simulink model "sampleModel2058"  (R2023a)
settings: Solver=VariableStepAuto  StartTime=0.0  StopTime=10.0  RelTol=1e-3
libraries: hdlsllib x4, simulink x2
settings Model: Creator=user1  LastModifiedBy=user1

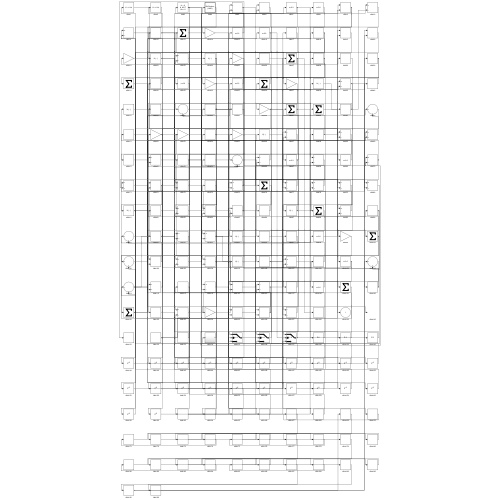
[thumbnail: Simulink's stored preview of the top-level diagram]
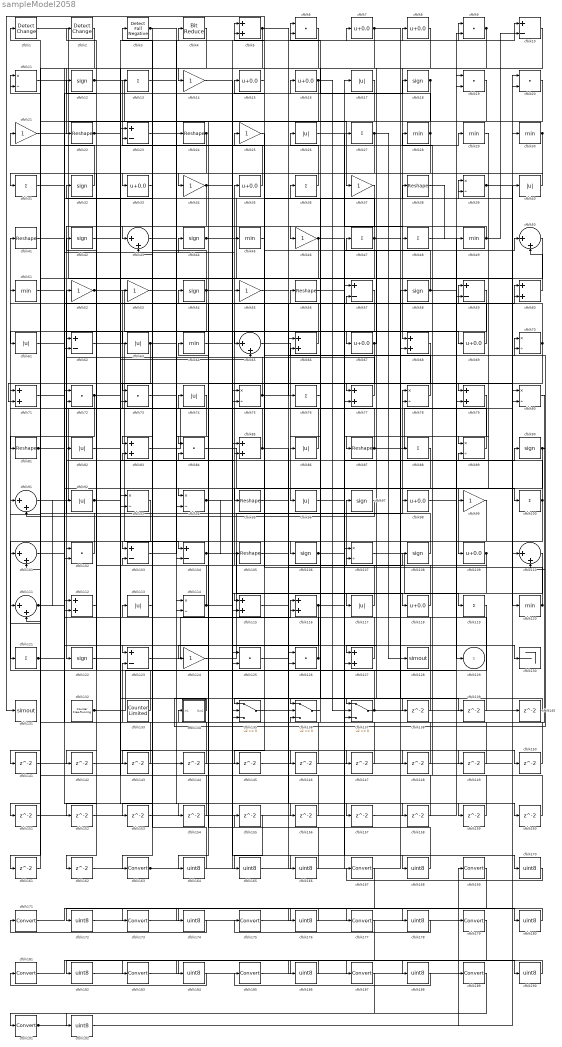
== system sampleModel2058 ==
  cfblk1 : simulink/Logic and Bit Operations/Detect Change  vinit=0  OutDataTypeStr=boolean
      settings: LibrarySourceBlock=|
      | hdlsllib/Logic and Bit
      | Operations/Detect
      | Change
  cfblk{10,23,57,59,62,103..104,123} (8 alike) : Sum  Inputs=+-
  cfblk{13,27,31,36,47..48,76,88,100,119,121} (11 alike) : Sum  Inputs=+
  cfblk{43,50,65,91,101,110..111} (7 alike) : Sum  Inputs=|++
  cfblk{6,9,19..20,72..73,84,102,125..126} (10 alike) : DotProduct  OutDataTypeStr=Inherit: Inherit via internal rule
  cfblk{22,24,38,41,56,81,87,95,105} (9 alike) : Reshape
  cfblk{12,18,32,42,44,54,58,90,97,106,108,122} (12 alike) : Signum
  cfblk{11,39,70,75,78,80,89,93..94,107,114} (11 alike) : Product  Inputs=*/  RndMeth=Zero  SaturateOnIntegerOverflow=on
  cfblk{7..8,15..16,33,35,67,69,98,109,118} (11 alike) : Bias  Bias=0.0  SaturateOnIntegerOverflow=off
  cfblk{5,60,66,68,71,77,79,83,85,112,115..116,127} (13 alike) : Sum
  cfblk{17,26,40,61,63,74,82,86,92,96,113,117} (12 alike) : Abs  SaturateOnIntegerOverflow=off
  cfblk{28..30,45,49,51,64,120} (8 alike) : MinMax
  cfblk{14,21,25,34,37,46,52..53,55,99,124} (11 alike) : Gain
  cfblk128 : ToWorkspace  VariableName=simout  SaveFormat=Timeseries  SampleTime=-1
  cfblk130 : Terminator
  cfblk131 : ToWorkspace  VariableName=simout  SaveFormat=Timeseries  SampleTime=-1
  cfblk132 : hdlsllib/Sources/Counter Free-Running  NumBits=16  tsamp=-1
  cfblk133 : hdlsllib/Sources/Counter Limited  uplimit=7  tsamp=-1
  cfblk134 : Subsystem
      settings: LibrarySourceBlock=|
      | hdlsllib/Ports &
      | Subsystems/Subsystem
  cfblk135 : Switch  SaturateOnIntegerOverflow=off  InputSameDT=off
  cfblk136 : Switch  SaturateOnIntegerOverflow=off  InputSameDT=off
  cfblk137 : Switch  SaturateOnIntegerOverflow=off  InputSameDT=off
  cfblk{138..162} (25 alike) : Delay  SampleTime=1
  cfblk{163,167,169,171,173,175,177,179,181,183,185,187,189,191} (14 alike) : DataTypeConversion  SaturateOnIntegerOverflow=off  RndMeth=Floor
  cfblk{164..166,168,170,172,174,176,178,180,182,184,186,188,190,192} (16 alike) : DataTypeConversion  OutDataTypeStr=uint8  SaturateOnIntegerOverflow=off  RndMeth=Floor
  cfblk2 : simulink/Logic and Bit Operations/Detect Change  vinit=0  OutDataTypeStr=boolean
      settings: LibrarySourceBlock=|
      | hdlsllib/Logic and Bit
      | Operations/Detect
      | Change
  cfblk3 : hdlsllib/Logic and Bit Operations/Detect Fall Negative  vinit=0  OutDataTypeStr=boolean
  cfblk4 : hdlsllib/Logic and Bit Operations/Bit Reduce  mode=AND
  cfblk129 : Outport  VectorParamsAs1DForOutWhenUnconnected=off
  wires:
  cfblk37/1 -> cfblk122/1
  cfblk100/1 -> cfblk102/1, cfblk12/1, cfblk164/1
  cfblk5/1 -> cfblk14/1, cfblk77/1
  cfblk62/1 -> cfblk104/1
  cfblk117/1 -> cfblk35/1
  cfblk25/1 -> cfblk95/1
  cfblk52/1 -> cfblk69/1, cfblk152/1
  cfblk12/1 -> cfblk37/1, cfblk65/2
  cfblk119/1 -> cfblk41/1
  cfblk86/1 -> cfblk15/1
  cfblk89/1 -> cfblk53/1
  cfblk126/1 -> cfblk54/1, cfblk43/2
  cfblk8/1 -> cfblk68/1
  cfblk93/1 -> cfblk121/1
  cfblk113/1 -> cfblk163/1
  cfblk118/1 -> cfblk97/1
  cfblk102/1 -> cfblk52/1
  cfblk57/1 -> cfblk67/1
  cfblk96/1 -> cfblk50/1
  cfblk40/1 -> cfblk34/1
  cfblk84/1 -> cfblk109/1
  cfblk77/1 -> cfblk62/1
  cfblk124/1 -> cfblk78/1
  cfblk123/1 -> cfblk116/1
  cfblk65/1 -> cfblk96/1
  cfblk121/1 -> cfblk56/1, cfblk44/1
  cfblk101/1 -> cfblk16/1
  cfblk51/1 -> cfblk63/1
  cfblk22/1 -> cfblk148/1, cfblk149/1
  cfblk66/1 -> cfblk51/1
  cfblk103/1 -> cfblk59/1
  cfblk21/1 -> cfblk129/1
  cfblk76/1 -> cfblk136/1
  cfblk94/1 -> cfblk105/1, cfblk10/1, cfblk147/1
  cfblk20/1 -> cfblk103/1
  cfblk107/1 -> cfblk119/1
  cfblk114/1 -> cfblk2/1, cfblk150/1
  cfblk115/1 -> cfblk108/1
  cfblk87/1 -> cfblk40/1, cfblk36/1
  cfblk18/1 -> cfblk124/1, cfblk115/2
  cfblk35/1 -> cfblk13/1
  cfblk15/1 -> cfblk131/1
  cfblk1/1 -> cfblk88/1
  cfblk32/1 -> cfblk21/1
  cfblk46/1 -> cfblk101/1, cfblk80/2, cfblk39/1
  cfblk61/1 -> cfblk38/1
  cfblk91/1 -> cfblk68/2
  cfblk85/1 -> cfblk11/1, cfblk158/1
  cfblk60/1 -> cfblk50/2
  cfblk78/1 -> cfblk55/1
  cfblk54/1 -> cfblk32/1, cfblk79/2, cfblk83/1
  cfblk29/1 -> cfblk99/1
  cfblk16/1 -> cfblk31/1, cfblk137/2
  cfblk72/1 -> cfblk111/2, cfblk4/1
  cfblk34/1 -> cfblk6/1, cfblk114/2
  cfblk90/1 -> cfblk112/2, cfblk110/2
  cfblk127/1 -> cfblk82/1
  cfblk81/1 -> cfblk29/1, cfblk45/1
  cfblk38/1 -> cfblk49/1
  cfblk120/1 -> cfblk25/1, cfblk28/1
  cfblk70/1 -> cfblk3/1, cfblk137/1
  cfblk19/1 -> cfblk102/2
  cfblk7/1 -> cfblk46/1, cfblk139/1
  cfblk88/1 -> cfblk106/1
  cfblk98/1 -> cfblk90/1
  cfblk27/1 -> cfblk86/1, cfblk128/1, cfblk75/2
  cfblk112/1 -> cfblk42/1
  cfblk111/1 -> cfblk74/1, cfblk92/1, cfblk157/1
  cfblk83/1 -> cfblk27/1
  cfblk135/1 -> cfblk107/2
  cfblk36/1 -> cfblk26/1
  cfblk41/1 -> cfblk18/1
  cfblk28/1 -> cfblk94/1, cfblk73/2, cfblk6/2
  cfblk80/1 -> cfblk134/1(In1)
  cfblk9/1 -> cfblk93/2, cfblk62/2
  cfblk106/1 -> cfblk98/1, cfblk60/2
  cfblk53/1 -> cfblk24/1
  cfblk24/1 -> cfblk61/1, cfblk161/1
  cfblk110/1 -> cfblk126/2
  cfblk63/1 -> cfblk9/1, cfblk8/1, cfblk71/2
  cfblk108/1 -> cfblk71/1
  cfblk17/1 -> cfblk81/1
  cfblk31/1 -> cfblk123/1
  cfblk134/1(Out1) -> cfblk70/1
  cfblk133/1 -> cfblk91/1
  cfblk33/1 -> cfblk73/1
  cfblk97/1 -> cfblk91/2
  cfblk75/1 -> cfblk23/2, cfblk70/2
  cfblk104/1 -> cfblk117/1, cfblk118/1
  cfblk3/1 -> cfblk77/2, cfblk143/1, cfblk146/1
  cfblk49/1 -> cfblk43/1, cfblk10/2
  cfblk74/1 -> cfblk94/2
  cfblk69/1 -> cfblk11/2
  cfblk39/1 -> cfblk120/1, cfblk89/1
  cfblk6/1 -> cfblk22/1
  cfblk132/1 -> cfblk19/1, cfblk85/1
  cfblk105/1 -> cfblk60/1
  cfblk55/1 -> cfblk76/1
  cfblk50/1 -> cfblk127/1
  cfblk26/1 -> cfblk48/1
  cfblk92/1 -> cfblk130/1, cfblk85/2
  cfblk43/1 -> cfblk104/2
  cfblk44/1 -> cfblk30/1, cfblk80/1, cfblk39/2
  cfblk79/1 -> cfblk127/2
  cfblk67/1 -> cfblk84/1, cfblk47/1
  cfblk11/1 -> cfblk114/1
  cfblk116/1 -> cfblk125/2, cfblk89/2
  cfblk10/1 -> cfblk87/1
  cfblk125/1 -> cfblk57/2
  cfblk4/1 -> cfblk33/1
  cfblk48/1 -> cfblk100/1
  cfblk137/1 -> cfblk72/2, cfblk20/1
  cfblk58/1 -> cfblk19/2, cfblk5/2
  cfblk42/1 -> cfblk79/1
  cfblk109/1 -> cfblk135/3, cfblk103/2
  cfblk45/1 -> cfblk115/1
  cfblk136/1 -> cfblk66/2
  cfblk47/1 -> cfblk59/2, cfblk5/1, cfblk162/1
  cfblk23/1 -> cfblk7/1
  cfblk30/1 -> cfblk65/1, cfblk142/1
  cfblk82/1 -> cfblk138/1
  cfblk138/1 -> cfblk112/1
  cfblk139/1 -> cfblk23/1
  cfblk140/1 -> cfblk135/1
  cfblk59/1 -> cfblk141/1
  cfblk141/1 -> cfblk107/1
  cfblk142/1 -> cfblk110/1
  cfblk143/1 -> cfblk123/2
  cfblk13/1 -> cfblk144/1
  cfblk144/1 -> cfblk1/1
  cfblk68/1 -> cfblk145/1
  cfblk145/1 -> cfblk136/2
  cfblk146/1 -> cfblk83/2
  cfblk147/1 -> cfblk66/1
  cfblk148/1 -> cfblk72/1
  cfblk149/1 -> cfblk136/3
  cfblk150/1 -> cfblk116/2
  cfblk2/1 -> cfblk151/1
  cfblk151/1 -> cfblk57/1
  cfblk152/1 -> cfblk137/3
  cfblk99/1 -> cfblk153/1
  cfblk153/1 -> cfblk125/1
  cfblk71/1 -> cfblk154/1
  cfblk154/1 -> cfblk111/1
  cfblk122/1 -> cfblk156/1
  cfblk156/1 -> cfblk135/2
  cfblk157/1 -> cfblk9/2
  cfblk158/1 -> cfblk84/2
  cfblk73/1 -> cfblk159/1
  cfblk159/1 -> cfblk78/2
  cfblk95/1 -> cfblk160/1
  cfblk160/1 -> cfblk93/1
  cfblk161/1 -> cfblk101/2
  cfblk162/1 -> cfblk75/1
  cfblk163/1 -> cfblk58/1, cfblk17/1
  cfblk164/1 -> cfblk113/1
  cfblk155/1 -> cfblk165/1
  cfblk165/1 -> cfblk126/1
  cfblk14/1 -> cfblk166/1
  cfblk166/1 -> cfblk155/1
  cfblk56/1 -> cfblk168/1
  cfblk168/1 -> cfblk64/1
  cfblk64/1 -> cfblk170/1
  cfblk170/1 -> cfblk167/1
  cfblk167/1 -> cfblk172/1
  cfblk172/1 -> cfblk169/1
  cfblk169/1 -> cfblk174/1
  cfblk174/1 -> cfblk171/1
  cfblk171/1 -> cfblk176/1
  cfblk176/1 -> cfblk173/1
  cfblk173/1 -> cfblk178/1
  cfblk178/1 -> cfblk175/1
  cfblk175/1 -> cfblk180/1
  cfblk180/1 -> cfblk177/1
  cfblk177/1 -> cfblk182/1
  cfblk182/1 -> cfblk179/1
  cfblk179/1 -> cfblk184/1
  cfblk184/1 -> cfblk181/1
  cfblk181/1 -> cfblk186/1
  cfblk186/1 -> cfblk183/1
  cfblk183/1 -> cfblk188/1
  cfblk188/1 -> cfblk185/1
  cfblk189/1 -> cfblk191/1
  cfblk185/1 -> cfblk190/1
  cfblk190/1 -> cfblk187/1
  cfblk191/1 -> cfblk140/1, cfblk20/2
  cfblk187/1 -> cfblk192/1
  cfblk192/1 -> cfblk189/1

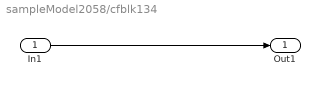
== system sampleModel2058/cfblk134 ==
  In1 : Inport
  Out1 : Outport
  wires:
  In1/1 -> Out1/1
